simulink model "NewModuleTry_cs"  (Simulink 8.4)
settings: Solver=ode5  SolverMode=SingleTasking  StartTime=0.0  StopTime=inf  FixedStep=1/100  RelTol=1e-3
model workspace (MAT data in the model file):
  mbox_table : struct (value not decoded)
  model_closed = 0
  sim_status : num (value not decoded)
PreLoadFcn:
  | mbxruntime.callbacks.PreLoadFcn(bdroot);
PostLoadFcn:
  | mbxruntime.callbacks.PostLoadFcn(bdroot);
InitFcn:
  | mbxruntime.callbacks.InitFcn(bdroot);
StartFcn:
  | mbxruntime.callbacks.StartFcn(bdroot);
StopFcn:
  | mbxruntime.callbacks.StopFcn(bdroot);
undefined symbols (not defined in the file or in its folder): dfreq, gray, InitImageOutputDir, Rec, SDTV, strel
libraries: simulink x41, PreScanSimulinkLibrary x15, visiontextngfix x15, simulink_extras x12, visionconversions x3, PreScanUsefulBlocks x3, visionsinks x2, visionstatistics x1, visionmorphops x1, visionanalysis x1, simulink_need_slupdate x1
(part 1 of 7)
CloseFcn:
  | mbxruntime.callbacks.CloseFcn(bdroot);
settings Model: Creator=PRESCAN  LastModifiedBy=vj-admin
settings OptimizationCC: InitFltsAndDblsToZero=on
settings DebuggingCC: SaveWithParameterizedLinksMsg=none  SignalResolutionControl=TryResolveAllWithWarning  SolverPrmCheckMsg=none  MultiTaskDSMMsg=warning  MultiTaskCondExecSysMsg=none
settings ModelReferenceCC: UpdateModelReferenceTargets=IfOutOfDate
settings SFSimCC: SimParseCustomCode=off
settings SFSimCC: SimCustomHeaderCode=|
  | #include "prescan_collisiondetection_data.h"
  | #include "prescan.h"
  | #include "prescan_platform.h"
  | #include "prescan_v2x_data.h"
settings RTWCC: IncludeERTFirstTime=on
settings GRTTargetCC: TargetFcnLib=ansi_tfl_tmw.mat

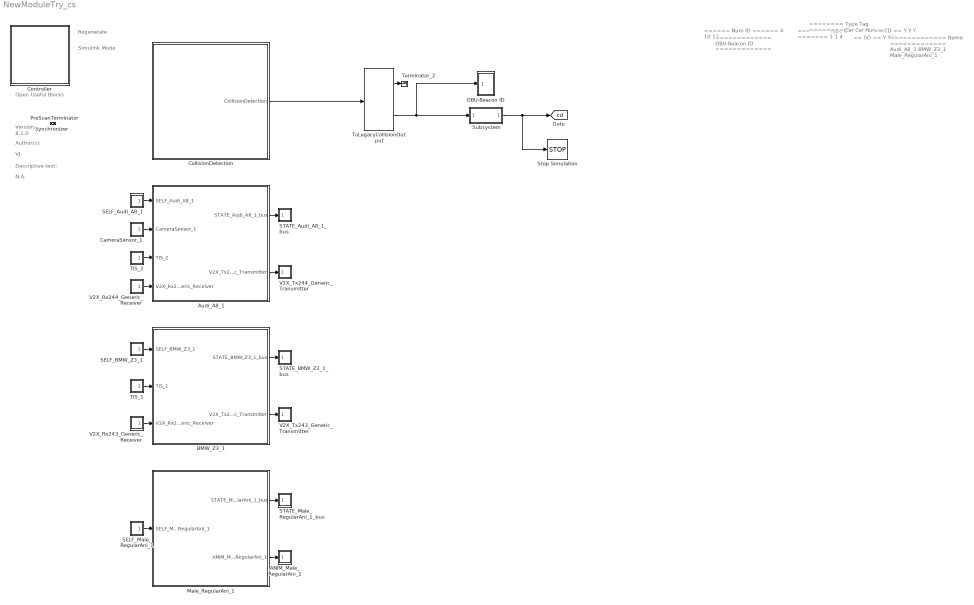
== system NewModuleTry_cs ==
  note: Regenerate
  note: Simulink Mode
  note: Open Useful Blocks
  note: 8.1.0
  note: Version:
  note: Author(s):
  note: VJ
  note: Descriptive text:
  note: N.A.
  note: ======
      | Num ID
      | ======
      | 4
      | 10
      | 11
  note: =============
      | OBU-Beacon ID
      | =============
  note: =======
      | Type ID
      | =======
      | 1
      | 1
      | 4
  note: ========
      | Type Tag
      | ========
      | Car
      | Car
      | Human
  note: ==
      | SD
      | ==
      | Y
      | Y
      | Y
  note: ==
      | CD
      | ==
      | Y
      | Y
      | Y
  note: =============
      | Name
      | =============
      | Audi_A8_1
      | BMW_Z3_1
      | Male_RegularAni_1
  ANIM_Male_RegularAni_1 : Subsystem  Tag=actuator/AnimationOutport  Priority=0  LoadFcn=load('PreScanAnimActuatorData.mat')  Variant=on  OverrideUsingVariant=on  mask(PreScan Sink Block: State Animation){}
      mask help: The Human Animation port allows the human to walk, run or bend
      settings: OpenFcn=open_system([gcb '/ENABLED/Actuator'],'mask')
      mask Help: eval('openHelp(239)')
      mask Display: image(imread('HumanAnimated.jpg'))
  Audi_A8_1 : Subsystem  Tag=WorldObjectSubSystem  InitFcn=UniqueId = '58';  Variant=on  OverrideUsingVariant=on
      mask init:
      | imagePath=which('Audi_A8.jpg');
      settings: OpenFcn=open_system([gcb '/ENABLED'])
      mask Display: image(imread(imagePath));color('white');text(0,0,' ID=4\n')
  BMW_Z3_1 : Subsystem  Tag=WorldObjectSubSystem  InitFcn=UniqueId = '59';  Variant=on  OverrideUsingVariant=on
      mask init:
      | imagePath=which('BMW_Z3.jpg');
      settings: OpenFcn=open_system([gcb '/ENABLED'])
      mask Display: image(imread(imagePath));color('white');text(0,0,' ID=10\n')
  CameraSensor_1 : Subsystem  Tag=sensor/Camera/CameraSensor  Priority=3  Variant=on  OverrideUsingVariant=on  mask(PreScan Source Block: Camera Sensor){}
      mask help: The Camera Sensor provides a color or monochrome image.
      settings: OpenFcn=open_system([gcb '/ENABLED/Sensor'],'mask')
      mask Help: eval('openHelp(457)')
      mask Display: image(imread('CameraSensor.png'))
  CollisionDetection : Subsystem  Tag=sensor/CollisionDetection  Priority=3  LoadFcn=load('PrescanCollisionDetectionData.mat');load('PrescanCollisionDetectionMessage.mat')  Variant=on  OverrideUsingVariant=on  mask(PreScan Source Block: CollisionDetection){}
      mask help: Collision Detection can be used to detect collisions between PreScan components. For Collision Detection the actual component shape is taken into account, so it is not a bounding box approach.
      settings: OpenFcn=open_system([gcb '/ENABLED/Sensor'],'mask')
      mask Help: eval('openHelp(811)')
      mask Display: image(imread('crash.jpg'))
  Controller : Subsystem  Description=A11229525821A304D5856380C190912EEAC74B144EF439124D49D263F028B97E  Priority=-1  LoadFcn=load PreScanControllerData  mask(PreScan Simulation Controller){prescanversion='8.1.0', ModelReferencing=off, TimeStep=1/100, ControlMode=0, PreScanExecutionMode=on, ControllerCount=0, ControllerIndex=0, ControllerOptions=''}
      mask prompts: prescanversion "PreScan Version"; ModelReferencing "Use Model Referencing"; TimeStep "Upload Period [s]"; ControlMode "Control Mode"; PreScanExecutionMode "Execution Mode"; ControllerCount "Controller Count"; ControllerIndex "Controller Index"; ControllerOptions "Controller Options"
      mask help:
      | Please do not remove this block from the compilation sheet,
      | as it connects the model to the PreScan environment.
      mask init:
      | model = bdroot(gcb);
      | ExperimentFile = mbxruntime.findExperimentFile(model);
      | 
      | [d1, d2, d3, prescandata] = prescan_Settings();
      | ModelDepo = fullfile(prescandata,'ModelDepo'); 
      | 
      | RTmode = 0;
      | actors = find_system(model,'SearchDepth', 1,'LookUnderMasks', 'all','Tag','WorldObjectSubSystem');
      | for ii=1:length(actors)
      |     actormode = get_param(actors{ii},'OverrideUsingVariant');
      |     if strcmpi(actormode,'off')
      |         RTmode = 1;
      |     end
      | end
      | 
      | SimulationMode = get_param(bdroot,'SimulationMode');
      | if strcmp(SimulationMode, 'rapid-accelerator')
      |     SimulationMode = 'external';
      | end
      | TargetName = get_param(bdroot,'SystemTargetFile');
      settings: ModelCloseFcn=assignin('base',['model_closed_' bdroot],true);
      mask Help: eval('openHelp(812)')
      mask Display: image(imread('prescanlogo.ico'))
  Male_RegularAni_1 : Subsystem  Tag=WorldObjectSubSystem  InitFcn=UniqueId = '60';  Variant=on  OverrideUsingVariant=on
      mask init:
      | imagePath=which('Male_RegularAni.jpg');
      settings: OpenFcn=open_system([gcb '/ENABLED'])
      mask Display: image(imread(imagePath));color('white');text(0,0,' ID=11\n')
  OBU-Beacon ID : Subsystem  Tag=Scope Collision Detections
      settings: DeleteFcn=PreScanBlockDeleteFcn;
      settings: OpenFcn=|
      | blockname=[get_param(gcb,'Parent'),'/',get_param(gcb,'Name')];
      | subblockname=[blockname,'/Collision Detections'];
      | open_system(subblockname);
      | close_system(blockname);
      mask Display:
      | plot([0.5 9.5 9.5 0.5 0.5],[5 5 9 9 5])
      | plot(0,0)
      | plot(10,10)
      | text(0,1,'P+')
  PreScanTerminator : Subsystem  Tag=PreScanTerminator  Priority=999  LoadFcn=load PrescanTerminatorData  mask(PreScan Simulation Terminator){TimeStep=1/100}
      mask prompts: TimeStep "Upload Period [s]"
      mask help:
      | Please do not remove this block from the compilation sheet as it
      | connects the model to the PreScan environment.
      mask Help: eval('openHelp(812)')
      mask Display: image(imread('prescanlogo.ico'))
  SELF_Audi_A8_1 : Subsystem  Tag=sensor/SelfPort  Priority=3  LoadFcn=load('PreScanSelfSensorData.mat')  Variant=on  OverrideUsingVariant=on  mask(PreScan Source Block: SELF){}
      mask help:
      | The SELF port shows (state) information of the actor itself. The outputs are position in the experiment's axis system and the GPS coordinates, and the object's absolute velocity and compass heading.
      |
      | For more information, please click Help.
      settings: OpenFcn=open_system([gcb '/ENABLED/Sensor'],'mask')
      mask Help: eval('openHelp(462)')
      mask Display: image(imread('GPS.png'))
  SELF_BMW_Z3_1 : Subsystem  Tag=sensor/SelfPort  Priority=3  LoadFcn=load('PreScanSelfSensorData.mat')  Variant=on  OverrideUsingVariant=on  mask(PreScan Source Block: SELF){}
      mask help:
      | The SELF port shows (state) information of the actor itself. The outputs are position in the experiment's axis system and the GPS coordinates, and the object's absolute velocity and compass heading.
      |
      | For more information, please click Help.
      settings: OpenFcn=open_system([gcb '/ENABLED/Sensor'],'mask')
      mask Help: eval('openHelp(462)')
      mask Display: image(imread('GPS.png'))
  SELF_Male_RegularAni_1 : Subsystem  Tag=sensor/SelfPort  Priority=3  LoadFcn=load('PreScanSelfSensorData.mat')  Variant=on  OverrideUsingVariant=on  mask(PreScan Source Block: SELF){}
      mask help:
      | The SELF port shows (state) information of the actor itself. The outputs are position in the experiment's axis system and the GPS coordinates, and the object's absolute velocity and compass heading.
      |
      | For more information, please click Help.
      settings: OpenFcn=open_system([gcb '/ENABLED/Sensor'],'mask')
      mask Help: eval('openHelp(462)')
      mask Display: image(imread('GPS.png'))
  STATE_Audi_A8_1_bus : Subsystem  Tag=actuator/StatePort  Priority=0  LoadFcn=load('PreScanStateActuatorData.mat')  Variant=on  OverrideUsingVariant=on  mask(PreScan Sink Block: State){}
      mask help:
      | The Actor State contains a vector signal of size (9x1), containing the following signals:
      |
      | -  Position    	(x,y,z)             	[m]
      | -  Velocity    	(vx,vy,vz)         	[m/s]
      | -  Angles       	(Roll, Pitch, Yaw)	[rad]
      |
      | The Actor state is defined in the global axis system.
      | The state is superponed on the Initial position defined in the GUI.
      |
      | For more information, please click Help.
      settings: OpenFcn=open_system([gcb '/ENABLED/Actuator'],'mask')
      mask Help: eval('openHelp(222)')
      mask Display: image(imread('State.png'))
  STATE_BMW_Z3_1_bus : Subsystem  Tag=actuator/StatePort  Priority=0  LoadFcn=load('PreScanStateActuatorData.mat')  Variant=on  OverrideUsingVariant=on  mask(PreScan Sink Block: State){}
      mask help:
      | The Actor State contains a vector signal of size (9x1), containing the following signals:
      |
      | -  Position    	(x,y,z)             	[m]
      | -  Velocity    	(vx,vy,vz)         	[m/s]
      | -  Angles       	(Roll, Pitch, Yaw)	[rad]
      |
      | The Actor state is defined in the global axis system.
      | The state is superponed on the Initial position defined in the GUI.
      |
      | For more information, please click Help.
      settings: OpenFcn=open_system([gcb '/ENABLED/Actuator'],'mask')
      mask Help: eval('openHelp(222)')
      mask Display: image(imread('State.png'))
  STATE_Male_RegularAni_1_bus : Subsystem  Tag=actuator/StatePort  Priority=0  LoadFcn=load('PreScanStateActuatorData.mat')  Variant=on  OverrideUsingVariant=on  mask(PreScan Sink Block: State){}
      mask help:
      | The Actor State contains a vector signal of size (9x1), containing the following signals:
      |
      | -  Position    	(x,y,z)             	[m]
      | -  Velocity    	(vx,vy,vz)         	[m/s]
      | -  Angles       	(Roll, Pitch, Yaw)	[rad]
      |
      | The Actor state is defined in the global axis system.
      | The state is superponed on the Initial position defined in the GUI.
      |
      | For more information, please click Help.
      settings: OpenFcn=open_system([gcb '/ENABLED/Actuator'],'mask')
      mask Help: eval('openHelp(222)')
      mask Display: image(imread('State.png'))
  Stop Simulation : Stop
  Subsystem : Subsystem
      mask Display: fprintf('CD');
  Synchronizer : Subsystem  Tag=PreScanSynchronizer  Priority=1  LoadFcn=load PrescanSynchronizeData  mask(PreScan Simulation Core Block){TimeStep=1/100}
      mask prompts: TimeStep "Timestep [s]"
      mask help:
      | Please do not remove this block from the PreScan compilation sheet,
      | as it contains essential configuration parameters for a PreScan simulation.
      settings: DeleteFcn=PreScanBlockDeleteFcn;
      mask Display: image(imread('prescanlogo.ico'))
  TIS_1 : Subsystem  Tag=sensor/TIS  Priority=3  LoadFcn=load('PrescanScannerSensorData.mat');load('PrescanScannerSensorMessage.mat')  Variant=on  OverrideUsingVariant=on  mask(PreScan Source Block: Technology Independent Sensor (TIS)){}
      mask help:
      | The Technology Independent Sensor (TIS) provides a sensor with all sensor-related influence factors (like noise, drift and accuracy) without being technology specific (like radar and lidar). The TIS detects the closest point on the geometry of an object.
      |
      | For more information, please click Help.
      settings: OpenFcn=open_system([gcb '/ENABLED/Sensor'],'mask')
      mask Help: eval('openHelp(449)')
      mask Display: image(imread('TIS.png'))
  TIS_2 : Subsystem  Tag=sensor/TIS  Priority=3  LoadFcn=load('PrescanScannerSensorData.mat');load('PrescanScannerSensorMessage.mat')  Variant=on  OverrideUsingVariant=on  mask(PreScan Source Block: Technology Independent Sensor (TIS)){}
      mask help:
      | The Technology Independent Sensor (TIS) provides a sensor with all sensor-related influence factors (like noise, drift and accuracy) without being technology specific (like radar and lidar). The TIS detects the closest point on the geometry of an object.
      |
      | For more information, please click Help.
      settings: OpenFcn=open_system([gcb '/ENABLED/Sensor'],'mask')
      mask Help: eval('openHelp(449)')
      mask Display: image(imread('TIS.png'))
  Terminator_2 : Terminator
  ToLegacyCollisionOutput : PreScanUsefulBlocks/ToLegacyCollisionOutput
  V2X_Rx243_Generic_Receiver : Subsystem  Tag=sensor/plugin/sfun_V2X_Generic_Receiver  Priority=3  Variant=on  OverrideUsingVariant=on  mask(V2X Generic Receiver Block){}
      mask help: V2X Block receiving a Generic message
      settings: OpenFcn=open_system([gcb '/ENABLED/Sensor'],'mask')
      mask Help: eval('openHelp()')
      mask Display: image(imread('V2XR_grayscale.png'))
  V2X_Rx244_Generic_Receiver : Subsystem  Tag=sensor/plugin/sfun_V2X_Generic_Receiver  Priority=3  Variant=on  OverrideUsingVariant=on  mask(V2X Generic Receiver Block){}
      mask help: V2X Block receiving a Generic message
      settings: OpenFcn=open_system([gcb '/ENABLED/Sensor'],'mask')
      mask Help: eval('openHelp()')
      mask Display: image(imread('V2XR_grayscale.png'))
  V2X_Tx243_Generic_Transmitter : Subsystem  Tag=actuator/plugin/sfun_V2X_Generic_Transmitter  Priority=0  Variant=on  OverrideUsingVariant=on  mask(V2X Generic Transmitter Block){}
      mask help: V2X Block transmitting a Generic message
      settings: OpenFcn=open_system([gcb '/ENABLED/Actuator'],'mask')
      mask Help: eval('openHelp()')
      mask Display: image(imread('V2XT_grayscale.png'))
  V2X_Tx244_Generic_Transmitter : Subsystem  Tag=actuator/plugin/sfun_V2X_Generic_Transmitter  Priority=0  Variant=on  OverrideUsingVariant=on  mask(V2X Generic Transmitter Block){}
      mask help: V2X Block transmitting a Generic message
      settings: OpenFcn=open_system([gcb '/ENABLED/Actuator'],'mask')
      mask Help: eval('openHelp()')
      mask Display: image(imread('V2XT_grayscale.png'))
  tag scope: cd=global
  wires:
  CollisionDetection/1(CollisionDetection) -> ToLegacyCollisionOutput/1
  Subsystem/1(cd_out) -> Stop Simulation/1, [cd]
  ToLegacyCollisionOutput/2 -> Subsystem/1(cd_in), OBU-Beacon ID/1(In1)
  ToLegacyCollisionOutput/1 -> Terminator_2/1
  Audi_A8_1/1(STATE_Audi_A8_1_bus) -> STATE_Audi_A8_1_bus/1(STATE_Audi_A8_1_bus)
  SELF_Audi_A8_1/1(SELF_Audi_A8_1) -> Audi_A8_1/1(SELF_Audi_A8_1)
  CameraSensor_1/1(CameraSensor_1) -> Audi_A8_1/2(CameraSensor_1)
  TIS_2/1(TIS_2) -> Audi_A8_1/3(TIS_2)
  Audi_A8_1/2(V2X_Tx244_Generic_Transmitter) -> V2X_Tx244_Generic_Transmitter/1(V2X_Tx244_Generic_Transmitter)
  V2X_Rx244_Generic_Receiver/1(V2X_Rx244_Generic_Receiver) -> Audi_A8_1/4(V2X_Rx244_Generic_Receiver)
  BMW_Z3_1/1(STATE_BMW_Z3_1_bus) -> STATE_BMW_Z3_1_bus/1(STATE_BMW_Z3_1_bus)
  SELF_BMW_Z3_1/1(SELF_BMW_Z3_1) -> BMW_Z3_1/1(SELF_BMW_Z3_1)
  TIS_1/1(TIS_1) -> BMW_Z3_1/2(TIS_1)
  BMW_Z3_1/2(V2X_Tx243_Generic_Transmitter) -> V2X_Tx243_Generic_Transmitter/1(V2X_Tx243_Generic_Transmitter)
  V2X_Rx243_Generic_Receiver/1(V2X_Rx243_Generic_Receiver) -> BMW_Z3_1/3(V2X_Rx243_Generic_Receiver)
  Male_RegularAni_1/1(STATE_Male_RegularAni_1_bus) -> STATE_Male_RegularAni_1_bus/1(STATE_Male_RegularAni_1_bus)
  Male_RegularAni_1/2(ANIM_Male_RegularAni_1) -> ANIM_Male_RegularAni_1/1(ANIM_Male_RegularAni_1)
  SELF_Male_RegularAni_1/1(SELF_Male_RegularAni_1) -> Male_RegularAni_1/1(SELF_Male_RegularAni_1)

== system NewModuleTry_cs/ANIM_Male_RegularAni_1 ==
  ANIM_Male_RegularAni_1 : Inport  Tag=inport/AnimationOutport  OutDataTypeStr=Bus: PRESCAN_ANIMACTUATORDATA  PortDimensions=1  SampleTime=1/100  BusOutputAsStruct=on
  DISABLED : Subsystem  VariantControl=off
  ENABLED : Subsystem  VariantControl=on

== system NewModuleTry_cs/Audi_A8_1 ==
  SELF_Audi_A8_1 : Inport  Tag=inport/SelfPort  OutDataTypeStr=Bus: PRESCAN_SELFSENSORDATA  PortDimensions=1  SampleTime=1/100  BusOutputAsStruct=on
  CameraSensor_1 : Inport  Tag=inport/Camera/CameraSensor  Port=2  OutDataTypeStr=uint8  SampleTime=1/50  BusOutputAsStruct=on
  TIS_2 : Inport  Tag=inport/TIS  Port=3  OutDataTypeStr=Bus: PRESCAN_SCANNERSENSOR_MESSAGE  PortDimensions=1  SampleTime=1/25  BusOutputAsStruct=on
  V2X_Rx244_Generic_Receiver : Inport  Tag=inport/plugin/sfun_V2X_Generic_Receiver  Port=4  BusOutputAsStruct=on
  DISABLED : Subsystem  VariantControl=off
  ENABLED : Subsystem  VariantControl=on
  STATE_Audi_A8_1_bus : Outport  Tag=outport/StatePort  OutDataTypeStr=Bus: PRESCAN_STATEACTUATORDATA  PortDimensions=1  SampleTime=1/100
  V2X_Tx244_Generic_Transmitter : Outport  Tag=outport/plugin/sfun_V2X_Generic_Transmitter  Port=2

== system NewModuleTry_cs/BMW_Z3_1 ==
  SELF_BMW_Z3_1 : Inport  Tag=inport/SelfPort  OutDataTypeStr=Bus: PRESCAN_SELFSENSORDATA  PortDimensions=1  SampleTime=1/100  BusOutputAsStruct=on
  TIS_1 : Inport  Tag=inport/TIS  Port=2  OutDataTypeStr=Bus: PRESCAN_SCANNERSENSOR_MESSAGE  PortDimensions=1  SampleTime=1/25  BusOutputAsStruct=on
  V2X_Rx243_Generic_Receiver : Inport  Tag=inport/plugin/sfun_V2X_Generic_Receiver  Port=3  BusOutputAsStruct=on
  DISABLED : Subsystem  VariantControl=off
  ENABLED : Subsystem  VariantControl=on
  STATE_BMW_Z3_1_bus : Outport  Tag=outport/StatePort  OutDataTypeStr=Bus: PRESCAN_STATEACTUATORDATA  PortDimensions=1  SampleTime=1/100
  V2X_Tx243_Generic_Transmitter : Outport  Tag=outport/plugin/sfun_V2X_Generic_Transmitter  Port=2

== system NewModuleTry_cs/CameraSensor_1 ==
  DISABLED : Subsystem  VariantControl=off
  ENABLED : Subsystem  VariantControl=on
  CameraSensor_1 : Outport  Tag=outport/Camera/CameraSensor  OutDataTypeStr=uint8  SampleTime=1/50

== system NewModuleTry_cs/CollisionDetection ==
  DISABLED : Subsystem  VariantControl=off
  ENABLED : Subsystem  VariantControl=on
  CollisionDetection : Outport  Tag=outport/CollisionDetection  OutDataTypeStr=Bus: PRESCAN_COLLISIONDETECTION_MESSAGE  PortDimensions=1  SampleTime=1/100

== system NewModuleTry_cs/Controller ==
  Terminator : Terminator
  sfun_Controller : S-Function  FunctionName=sfun_Controller  Parameters=SParameter1, SParameter2, SParameter3, SParameter4, SParameter5, SParameter6, SParameter7, SParameter8, SParameter9, SParameter10, SampleTime  EnableBusSupport=off  mask(Legacy Function){SFunctionSpec=void prescan_outputFcn(void** work1, PRESCAN_CONTROLLERDATA y1[1]), SParameter1=uint8([ExperimentFile 0]), SParameter2=uint8([ModelDepo 0]), SParameter3=uint8([ControllerOptions 0]), SParameter4=RTmode, SParameter5=PreScanExecutionMode, SParameter6=ControlMode, SParameter7=ControllerCount, SParameter8=ControllerIndex, SParameter9=uint8([SimulationMode 0]), SParameter10=uint8([TargetName 0]), SampleTime=TimeStep, ShowSpec=on}
      mask prompts: SParameter1 "P1:"; SParameter2 "P2:"; SParameter3 "P3:"; SParameter4 "P4:"; SParameter5 "P5:"; SParameter6 "P6:"; SParameter7 "P7:"; SParameter8 "P8:"; SParameter9 "P9:"; SParameter10 "P10:"; SampleTime "Sample time (-1 for inherited):"; ShowSpec "Display function specification"
      mask help:
      | This block allows you to call the legacy functions specified by the following Legacy Code Tool definition:
      | def.SFunctionName = 'sfun_Controller';
      | def.OutputFcnSpec = 'void prescan_outputFcn(void** work1, PRESCAN_CONTROLLERDATA y1[1])';
      | def.StartFcnSpec = 'void prescan_startFcn(void ** work1, uint8 p1[], uint8 p2[], uint8 p3[], double p4, double p5, double p6, double p7, double p8, uint8 p9[], uint8 p10[])';
      | def.TerminateFcnSpec = 'void prescan_terminateFcn(void** work1)';
      | def.HeaderFiles = {'prescan_controller_data.h', 'prescan_SFunLibrary.h', 'prescan_LogHandler.h', 'prescan_CreateLogHandler.h', 'prescan_ErrorHandler.h', 'prescan_CreateErrorHandler.h', 'prescan_modify.h', 'ModuleDLL.h'};
      | def.SourceFiles = {'prescan_MexLogHandler.cpp', 'prescan_SimStructErrorHandler.cpp', 'prescan_LogHandler.cpp', 'prescan_ErrorHandler.cpp', 'prescan_Modify.cpp'};
      | def.HostLibFiles = {'sensorinterfaced.lib'};
      | def.TargetLibFiles = {'sensorinterfaced.so'};
      | def.IncPaths = {'.', 'C:\projects\prescan\rt_vislibrary\vis\..\pimp\include\sensors\InterfaceRTW'};
      | def.SrcPaths = {'C:\projects\prescan\rt_vislibrary\vis\..\pimp\include\sensors\InterfaceRTW', 'C:\projects\prescan\rt_vislibrary\vis\..\pimp\include\sensors\InterfaceRTW\ccurrt'};
      | def.LibPaths = {'C:\\projects\\prescan\\vislibrary_build\lib'};
      | def.SampleTime = 'parameterized';
      mask Help: <p>This block was generated automatically by the Legacy Code Tool. For detailed help on this tool, call<a href="matlab:legacy_code('help')"> legacy_code('help')</a>.</p>
      mask Callback ShowSpec:
      | if strcmp(get_param(gcbh, 'ShowSpec'), 'on')
      |   set_param(gcbh, 'MaskDisplay', sprintf('fprintf(''%s'');', get_param(gcbh, 'SFunctionSpec')));
      | else
      |   set_param(gcbh, 'MaskDisplay', sprintf('fprintf(''%s'');', get_param(gcbh, 'FunctionName')));
      | end
      mask Display: fprintf('void prescan_outputFcn(void** work1, PRESCAN_CONTROLLERDATA y1[1])');
  wires:
  sfun_Controller/1 -> Terminator/1

== system NewModuleTry_cs/Male_RegularAni_1 ==
  SELF_Male_RegularAni_1 : Inport  Tag=inport/SelfPort  OutDataTypeStr=Bus: PRESCAN_SELFSENSORDATA  PortDimensions=1  SampleTime=1/100  BusOutputAsStruct=on
  DISABLED : Subsystem  VariantControl=off
  ENABLED : Subsystem  VariantControl=on
  STATE_Male_RegularAni_1_bus : Outport  Tag=outport/StatePort  OutDataTypeStr=Bus: PRESCAN_STATEACTUATORDATA  PortDimensions=1  SampleTime=1/100
  ANIM_Male_RegularAni_1 : Outport  Tag=outport/AnimationOutport  Port=2  OutDataTypeStr=Bus: PRESCAN_ANIMACTUATORDATA  PortDimensions=1  SampleTime=1/100

== system NewModuleTry_cs/OBU-Beacon ID ==
  In1 : Inport
  Collision Detections : Scope  NumInputPorts=5
      settings: YMin=0~0~0~0~0  YMax=10~10~10~10~10  SaveName=ScopeData2
  Demux2 : Demux  Outputs=5
  wires:
  In1/1 -> Demux2/1
  Demux2/5 -> Collision Detections/5
  Demux2/4 -> Collision Detections/4
  Demux2/3 -> Collision Detections/3
  Demux2/2 -> Collision Detections/2
  Demux2/1 -> Collision Detections/1

== system NewModuleTry_cs/PreScanTerminator ==
  Terminator : Terminator
  sfun_Terminator : S-Function  FunctionName=sfun_Terminator  Parameters=SampleTime  EnableBusSupport=off  mask(Legacy Function){SFunctionSpec=void prescan_terminator_outputFcn(void ** work1, PRESCAN_TERMINATORDATA y1[1]), SampleTime=TimeStep, ShowSpec=on}
      mask prompts: SampleTime "Sample time (-1 for inherited):"; ShowSpec "Display function specification"
      mask help:
      | This block allows you to call the legacy functions specified by the following Legacy Code Tool definition:
      | def.SFunctionName = 'sfun_Terminator';
      | def.OutputFcnSpec = 'void prescan_terminator_outputFcn(void ** work1, PRESCAN_TERMINATORDATA y1[1])';
      | def.StartFcnSpec = 'void prescan_terminator_startFcn(void ** work1)';
      | def.TerminateFcnSpec = 'void prescan_terminator_terminateFcn(void ** work1)';
      | def.HeaderFiles = {'prescan_terminator_data.h'};
      | def.HostLibFiles = {'sensorinterfaced.lib'};
      | def.IncPaths = {'src', 'C:\prescandev\vislibrary\vis\..\pimp\include\sensors\InterfaceRTW'};
      | def.SrcPaths = {'src'};
      | def.LibPaths = {'C:\\prescandev\\vislibrary_build\lib'};
      | def.SampleTime = 'parameterized';
      | def.Options.language = 'C++';
      mask Help: <p>This block was generated automatically by the Legacy Code Tool. For detailed help on this tool, call<a href="matlab:legacy_code('help')"> legacy_code('help')</a>.</p>
      mask Callback ShowSpec:
      | if strcmp(get_param(gcbh, 'ShowSpec'), 'on')
      |   set_param(gcbh, 'MaskDisplay', sprintf('fprintf(''%s'');', get_param(gcbh, 'SFunctionSpec')));
      | else
      |   set_param(gcbh, 'MaskDisplay', sprintf('fprintf(''%s'');', get_param(gcbh, 'FunctionName')));
      | end
      mask Display: fprintf('void prescan_terminator_outputFcn(void ** work1, PRESCAN_TERMINATORDATA y1[1])');
  wires:
  sfun_Terminator/1 -> Terminator/1

== system NewModuleTry_cs/SELF_Audi_A8_1 ==
  DISABLED : Subsystem  VariantControl=off
  ENABLED : Subsystem  VariantControl=on
  SELF_Audi_A8_1 : Outport  Tag=outport/SelfPort  OutDataTypeStr=Bus: PRESCAN_SELFSENSORDATA  PortDimensions=1  SampleTime=1/100

== system NewModuleTry_cs/SELF_BMW_Z3_1 ==
  DISABLED : Subsystem  VariantControl=off
  ENABLED : Subsystem  VariantControl=on
  SELF_BMW_Z3_1 : Outport  Tag=outport/SelfPort  OutDataTypeStr=Bus: PRESCAN_SELFSENSORDATA  PortDimensions=1  SampleTime=1/100

== system NewModuleTry_cs/SELF_Male_RegularAni_1 ==
  DISABLED : Subsystem  VariantControl=off
  ENABLED : Subsystem  VariantControl=on
  SELF_Male_RegularAni_1 : Outport  Tag=outport/SelfPort  OutDataTypeStr=Bus: PRESCAN_SELFSENSORDATA  PortDimensions=1  SampleTime=1/100

== system NewModuleTry_cs/STATE_Audi_A8_1_bus ==
  STATE_Audi_A8_1_bus : Inport  Tag=inport/StatePort  OutDataTypeStr=Bus: PRESCAN_STATEACTUATORDATA  PortDimensions=1  SampleTime=1/100  BusOutputAsStruct=on
  DISABLED : Subsystem  VariantControl=off
  ENABLED : Subsystem  VariantControl=on

== system NewModuleTry_cs/STATE_BMW_Z3_1_bus ==
  STATE_BMW_Z3_1_bus : Inport  Tag=inport/StatePort  OutDataTypeStr=Bus: PRESCAN_STATEACTUATORDATA  PortDimensions=1  SampleTime=1/100  BusOutputAsStruct=on
  DISABLED : Subsystem  VariantControl=off
  ENABLED : Subsystem  VariantControl=on

== system NewModuleTry_cs/STATE_Male_RegularAni_1_bus ==
  STATE_Male_RegularAni_1_bus : Inport  Tag=inport/StatePort  OutDataTypeStr=Bus: PRESCAN_STATEACTUATORDATA  PortDimensions=1  SampleTime=1/100  BusOutputAsStruct=on
  DISABLED : Subsystem  VariantControl=off
  ENABLED : Subsystem  VariantControl=on

== system NewModuleTry_cs/Subsystem ==
  cd_in : Inport
  Integer Delay : Delay  DelayLength=1  InputProcessing=Inherited
  Logical Operator : Logic  AllPortsSameDT=off  OutDataTypeStr=boolean
  cd_out : Outport
  wires:
  cd_in/1 -> Integer Delay/1, Logical Operator/1
  Logical Operator/1 -> cd_out/1
  Integer Delay/1 -> Logical Operator/2

== system NewModuleTry_cs/Synchronizer ==
  Bus Selector1 : BusSelector  OutputSignals=FederateStopped
  Stop Simulation : Stop
  sfun_Synchronizer : S-Function  FunctionName=sfun_Synchronizer  Parameters=SampleTime  EnableBusSupport=off  mask(Legacy Function){SFunctionSpec=void prescan_synchronizer_outputFcn(void ** work1, PRESCAN_SYNCHRONIZEDATA y1[1]), SampleTime=TimeStep, ShowSpec=on}
      mask prompts: SampleTime "Sample time (-1 for inherited):"; ShowSpec "Display function specification"
      mask help:
      | This block allows you to call the legacy functions specified by the following Legacy Code Tool definition:
      | def.SFunctionName = 'sfun_Synchronizer';
      | def.OutputFcnSpec = 'void prescan_synchronizer_outputFcn(void ** work1, PRESCAN_SYNCHRONIZEDATA y1[1])';
      | def.StartFcnSpec = 'void prescan_synchronizer_startFcn(void ** work1)';
      | def.TerminateFcnSpec = 'void prescan_synchronizer_terminateFcn(void ** work1)';
      | def.HeaderFiles = {'prescan_synchronizer_data.h'};
      | def.HostLibFiles = {'sensorinterfaced.lib'};
      | def.IncPaths = {'src', 'C:\prescandev\vislibrary\vis\..\pimp\include\sensors\InterfaceRTW'};
      | def.SrcPaths = {'src'};
      | def.LibPaths = {'C:\\prescandev\\vislibrary_build\lib'};
      | def.SampleTime = 'parameterized';
      | def.Options.language = 'C++';
      mask Help: <p>This block was generated automatically by the Legacy Code Tool. For detailed help on this tool, call<a href="matlab:legacy_code('help')"> legacy_code('help')</a>.</p>
      mask Callback ShowSpec:
      | if strcmp(get_param(gcbh, 'ShowSpec'), 'on')
      |   set_param(gcbh, 'MaskDisplay', sprintf('fprintf(''%s'');', get_param(gcbh, 'SFunctionSpec')));
      | else
      |   set_param(gcbh, 'MaskDisplay', sprintf('fprintf(''%s'');', get_param(gcbh, 'FunctionName')));
      | end
      mask Display: fprintf('void prescan_synchronizer_outputFcn(void ** work1, PRESCAN_SYNCHRONIZEDATA y1[1])');
  wires:
  Bus Selector1/1 -> Stop Simulation/1  "<FederateStopped>"
  sfun_Synchronizer/1 -> Bus Selector1/1

== system NewModuleTry_cs/TIS_1 ==
  DISABLED : Subsystem  VariantControl=off
  ENABLED : Subsystem  VariantControl=on
  TIS_1 : Outport  Tag=outport/TIS  OutDataTypeStr=Bus: PRESCAN_SCANNERSENSOR_MESSAGE  PortDimensions=1  SampleTime=1/25

== system NewModuleTry_cs/TIS_2 ==
  DISABLED : Subsystem  VariantControl=off
  ENABLED : Subsystem  VariantControl=on
  TIS_2 : Outport  Tag=outport/TIS  OutDataTypeStr=Bus: PRESCAN_SCANNERSENSOR_MESSAGE  PortDimensions=1  SampleTime=1/25

== system NewModuleTry_cs/V2X_Rx243_Generic_Receiver ==
  DISABLED : Subsystem  VariantControl=off
  ENABLED : Subsystem  VariantControl=on
  V2X_Rx243_Generic_Receiver : Outport  Tag=outport/plugin/sfun_V2X_Generic_Receiver

== system NewModuleTry_cs/V2X_Rx244_Generic_Receiver ==
  DISABLED : Subsystem  VariantControl=off
  ENABLED : Subsystem  VariantControl=on
  V2X_Rx244_Generic_Receiver : Outport  Tag=outport/plugin/sfun_V2X_Generic_Receiver

== system NewModuleTry_cs/V2X_Tx243_Generic_Transmitter ==
  V2X_Tx243_Generic_Transmitter : Inport  Tag=inport/plugin/sfun_V2X_Generic_Transmitter  BusOutputAsStruct=on
  DISABLED : Subsystem  VariantControl=off
  ENABLED : Subsystem  VariantControl=on

== system NewModuleTry_cs/V2X_Tx244_Generic_Transmitter ==
  V2X_Tx244_Generic_Transmitter : Inport  Tag=inport/plugin/sfun_V2X_Generic_Transmitter  BusOutputAsStruct=on
  DISABLED : Subsystem  VariantControl=off
  ENABLED : Subsystem  VariantControl=on

== system NewModuleTry_cs/ANIM_Male_RegularAni_1/DISABLED ==
  ANIM_Male_RegularAni_1 : Inport  Tag=inport/AnimationOutport  OutDataTypeStr=Bus: PRESCAN_ANIMACTUATORDATA  PortDimensions=1  SampleTime=1/100  BusOutputAsStruct=on
  TRM1 : Terminator
  wires:
  ANIM_Male_RegularAni_1/1 -> TRM1/1

== system NewModuleTry_cs/ANIM_Male_RegularAni_1/ENABLED ==
  ANIM_Male_RegularAni_1 : Inport  Tag=inport/AnimationOutport  OutDataTypeStr=Bus: PRESCAN_ANIMACTUATORDATA  PortDimensions=1  SampleTime=1/100  BusOutputAsStruct=on
  Actuator : S-Function  FunctionName=sfun_AnimActuator  Parameters=UniqueID, TimeStep  EnableBusSupport=off  mask(PreScan Sink Block: State Animation){UniqueID=60, TimeStep=1/100}
      mask prompts: UniqueID "Auto-Assigned: Unique ID"; TimeStep "Auto-Assigned: Upload Period [s]"
      mask help: The Human Animation port allows the human to walk, run or bend
      mask Help: eval('openHelp(239)')
      mask Display: image(imread('HumanAnimated.jpg'))
  wires:
  ANIM_Male_RegularAni_1/1 -> Actuator/1

== system NewModuleTry_cs/Audi_A8_1/DISABLED ==
  SELF_Audi_A8_1 : Inport  Tag=inport/SelfPort  OutDataTypeStr=Bus: PRESCAN_SELFSENSORDATA  PortDimensions=1  SampleTime=1/100  BusOutputAsStruct=on
  CameraSensor_1 : Inport  Tag=inport/Camera/CameraSensor  Port=2  OutDataTypeStr=uint8  SampleTime=1/50  BusOutputAsStruct=on
  TIS_2 : Inport  Tag=inport/TIS  Port=3  OutDataTypeStr=Bus: PRESCAN_SCANNERSENSOR_MESSAGE  PortDimensions=1  SampleTime=1/25  BusOutputAsStruct=on
  V2X_Rx244_Generic_Receiver : Inport  Tag=inport/plugin/sfun_V2X_Generic_Receiver  Port=4  BusOutputAsStruct=on
  GND1 : Subsystem
  GND2 : Ground
  TRM{1..4} (4 alike) : Terminator
  STATE_Audi_A8_1_bus : Outport  Tag=outport/StatePort  OutDataTypeStr=Bus: PRESCAN_STATEACTUATORDATA  PortDimensions=1  SampleTime=1/100
  V2X_Tx244_Generic_Transmitter : Outport  Tag=outport/plugin/sfun_V2X_Generic_Transmitter  Port=2
  wires:
  SELF_Audi_A8_1/1 -> TRM1/1
  CameraSensor_1/1 -> TRM2/1
  TIS_2/1 -> TRM3/1
  V2X_Rx244_Generic_Receiver/1 -> TRM4/1
  GND1/1(bus) -> STATE_Audi_A8_1_bus/1
  GND2/1 -> V2X_Tx244_Generic_Transmitter/1

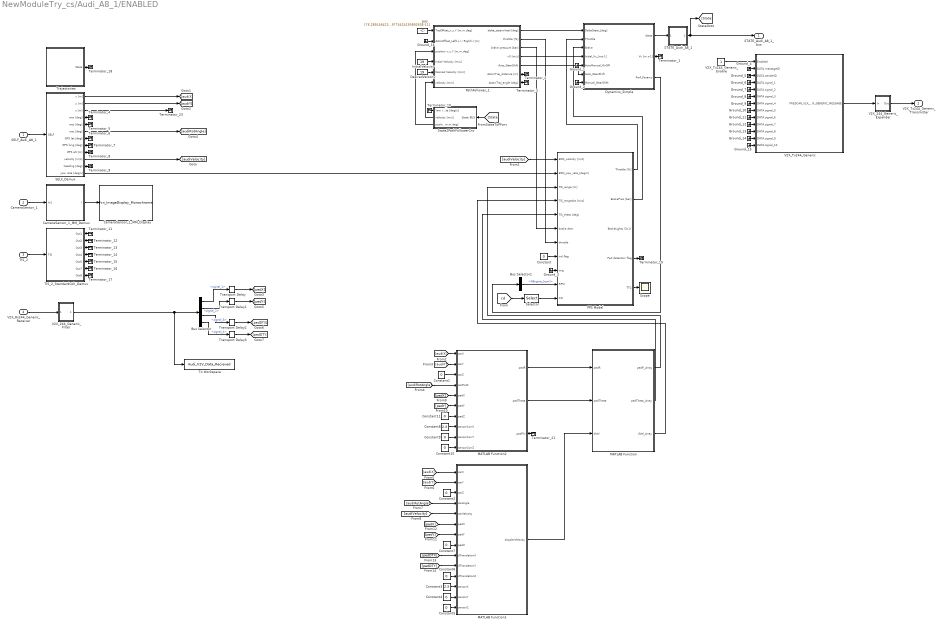
== system NewModuleTry_cs/Audi_A8_1/ENABLED ==
  SELF_Audi_A8_1 : Inport  Tag=inport/SelfPort  OutDataTypeStr=Bus: PRESCAN_SELFSENSORDATA  PortDimensions=1  SampleTime=1/100  BusOutputAsStruct=on
  CameraSensor_1 : Inport  Tag=inport/Camera/CameraSensor  Port=2  OutDataTypeStr=uint8  SampleTime=1/50  BusOutputAsStruct=on
  TIS_2 : Inport  Tag=inport/TIS  Port=3  OutDataTypeStr=Bus: PRESCAN_SCANNERSENSOR_MESSAGE  PortDimensions=1  SampleTime=1/25  BusOutputAsStruct=on
  V2X_Rx244_Generic_Receiver : Inport  Tag=inport/plugin/sfun_V2X_Generic_Receiver  Port=4  BusOutputAsStruct=on
  Bus Selector : BusSelector  OutputSignals=DATA.signal_1,DATA.signal_2,DATA.signal_3,DATA.signal_4
  Bus Selector1 : BusSelector  OutputSignals=NEngine_[rpm]
  CameraSensor_1_MM_Demux : Subsystem  Tag=demux/Camera/Monochrome  mask{SensorName=CameraSensor_1, hres=500, vres=375}
      mask prompts: SensorName "Sensor Name"; hres "Horizontal Resolution"; vres "Vertical Resolution"
      mask Help: eval('openHelp(457)')
      mask Display:
      | fprintf('MONO CAMERA:\n Monochrome\n %s \n %d x %d px',SensorName,hres,vres)
      | port_label('output',1,'I')
  CameraSensor_1_MM_Display : M-S-Function  Tag=CameraSensor_Monochrome_Display  InitFcn=InitImageOutputDir(gcb);  FunctionName=fcn_ImageDisplay_Monochrome  Parameters=SensorName EnableDisplay EnablePosition DisplayPosition FigureHandle SaveResults BitmapFormat TempOutputDir CameraType DataType  mask(PreScan Monochrome Display Block){SensorName=CameraSensor_1, EnableDisplay=on, EnablePosition=off, DisplayPosition=[10 10 500 375], FigureHandle=5801, SaveResults=off, Format=PNG, TempOutputDir=0, CameraType=Mono, DataType=uint8}
      mask prompts: SensorName "User Specified: Title of Display"; EnableDisplay "Active"; EnablePosition "Set Display window position"; DisplayPosition "Display window position [xpos ypos width height]"; FigureHandle "Unique handle"; SaveResults "Save results"; TempOutputDir "OutputDir"; CameraType "Camera Type"; DataType "Image Data Type"
      mask help: This block displays the Monochrome output of a PreScan camera sensor.
      mask init:
      | if EnableDisplay
      |     EnableString='';
      |     EnableColor='gray';
      | else
      |     EnableString='INACTIVE';
      |     EnableColor='red';
      | end
      | switch Format
      |     case 1
      |         BitmapFormat = 'png';
      |     case 2
      |         BitmapFormat = 'bmp';
      |     case 3
      |         BitmapFormat = 'jpg';
      | end
      | if CameraType==1
      |     CameraTypeName='MONO';
      |     PortNumber=0;
      | else
      |     CameraTypeName='STEREO';
      |     PortNumber=1;
      | end
      settings: CopyFcn=CopyFcnDisplay  DeleteFcn=PreScanBlockDeleteFcn;  ModelCloseFcn=fcn_ImageDisplay_ModelCloseFcn
      mask Help: eval('openHelp(457)')
      mask Callback EnablePosition:
      | MV=get_param(gcb,'MaskVisibilities');
      | if strcmp(get_param(gcb,'EnablePosition'),'on')
      |     MV{4}='on';
      | else
      |     MV{4}='off';
      | end
      | set_param(gcb,'MaskVisibilities',MV);
      | clear MV;
      mask TypeOptions Format: PNG | BMP | JPG
      mask TypeOptions CameraType: Mono | Stereo
      mask TypeOptions DataType: uint8 | single
      mask Display:
      | color(EnableColor);
      | fprintf('%s\n DISPLAY:\n Monochrome\n %s',EnableString,SensorName)
      | port_label('input',1,'I')
      | port_label('input',PortNumber+1,'I')
  Constant{,1..2,4..7,9..11} (10 alike) : Constant  Value=0
  Constant3 : Constant  Value=2.3
  Constant8 : Constant  Value=2.3
  DesiredVelocity : Constant  Tag=DesiredVelocity  Value=19
  Dynamics_Simple : Subsystem  Tag=Simple_Vehicle_Dynamics  mask(PreScan Block: Simple Dynamics){Migrate=on, TimeStep=1/100, ComputationMode=Continuous_Time}
      mask prompts: Migrate "Migrate. During migration this block will be replaced by a newer one."; TimeStep "Auto assigned: Time Step [s]"; ComputationMode "Computation mode:"
      mask help:
      | The Simple Dynamics Model is selected in the GUI to simulate vehicle dynamics behavior.
      |
      | The Simple Dynamics Model is completely open to the user. The parameters of this model can be set in the Simple Dynamics dialog in the GUI.
      |
      | For more information, please click Help.
      mask init:
      | p = SimpleDyn_pars;
      settings: DeleteFcn=PreScanBlockDeleteFcn;
      mask Help: eval('openHelp(220)')
      mask Display:
      | image(imread('SimpleDyn.png'))
      | port_label('input', 1, '{\delta}_S_t_ _e_e_r [deg]','texmode','on')
      | port_label('input', 2, 'Throttle [%]')
      | port_label('input', 3, 'Brake Pres [bar]')
      | port_label('input', 4, 'V_0 [ms-1]','texmode','on')
      | port_label('input', 5, 'Auto=[0]/Manual=[1]')
      | port_label('input', 6, 'Auto_GearShift')
      | port_label('input', 7, 'Manual_GearShift')
      | port_label('output', 1, 'State')
      | port_label('output', 2, 'Vx [ms-1]')
      | port_label('output', 3, 'Perf Params')
  Ground_{1..16} (16 alike) : Ground
  InitialVelocity : Constant  Tag=InitialVelocity  Value=19
  MATLAB Function : MATLAB Function  TreatAsAtomicUnit=on
  MATLAB Function1 : MATLAB Function  TreatAsAtomicUnit=on
  MATLAB Function2 : MATLAB Function  TreatAsAtomicUnit=on
  PPS Model : Subsystem  mask(PPS Model){MaxSpeed=70, MaxBrakePressure=150, BrakeDelay=100, LaneWidth=3.5, TISMaxRange=40, TISMaxTheta=60, TISfreq=25, TISdet=32, Camfreq=50, Mainfreq=100, DisplaySwitch=on, DisplayFreq=25, RadarSwitch=on, RadarFreq=25}
      mask prompts: MaxSpeed "Vehicle cut-off speed [km/h]"; MaxBrakePressure "Maximum value of braking pressure available [bar]"; BrakeDelay "Braking system delay [ms]"; LaneWidth "Lane width [m]"; TISMaxRange "TIS maximum range [m]"; TISMaxTheta "TIS maximum theta [deg]"; TISfreq "TIS frequency [Hz]"; TISdet "Max. number of Radar detected objects [-]"; Camfreq "Camera frequency [Hz]"; Mainfreq "Compilation sheet frequency [Hz]"; DisplaySwitch "Show EGO parameters visualization"; DisplayFreq "EGO parameters visualization frequency [Hz]"; RadarSwitch "Show radar visualization"; RadarFreq "Radar frequency [Hz]"
      mask help: PreScan Experiment and Pedestrian Protection System parameters
      mask Help: eval('openHelp(8130)')
      mask Callback DisplaySwitch:
      | en = get_param(gcb,'MaskEnables');
      | switch get_param(gcb, 'DisplaySwitch')
      |     case 'off'
      |         en{12} = 'off';
      |     case 'on'
      |         en{12} = 'on';
      | end
      | set_param(gcb,'MaskEnables',en);
      mask Callback RadarSwitch:
      | en = get_param(gcb,'MaskEnables');
      | switch get_param(gcb, 'RadarSwitch')
      |     case 'off'
      |         en{14} = 'off';
      |     case 'on'
      |         en{14} = 'on';
      | end
      | set_param(gcb,'MaskEnables',en);
  PathFollower_1 : Subsystem  Tag=pathFollower  mask(PreScan Block: Path Follower){Migrate=on, FileName='Trajectory_1.mat', TunableSteeringGain=1, XShifting_wrt_COG=0}
      mask prompts: Migrate "Migrate. During migration this block will be replaced by a newer one."; FileName "Trajectory Name"; TunableSteeringGain "TunableSteeringGain [-]"; XShifting_wrt_COG "XShifting_wrt_COG [m]"
      mask help:
      | The Path Follower Model is selected in the GUI to simulate driver behavior.
      |
      | For more information, please click Help.
      mask init:
      | load(['trajectories/',eval(FileName)])
      | traject=trajectory';
      | 
      | Traj_x=traject(:,2);
      | Traj_y=traject(:,3);
      | Traj_z=traject(:,4);
      | Traj_vx=traject(:,8);
      | Traj_vy=traject(:,9);
      | Traj_vz=traject(:,10);
      mask Help: eval('openHelp(232)')
  SELF_Demux : Subsystem  Tag=demux/SelfPort  mask(PreScan Demux Block:){}
      mask help:
      | The SELF port shows (state) information of the actor itself. The outputs are position in the experiment's axis system and the GPS coordinates, and the object's absolute velocity and compass heading.
      |
      | For more information, please click Help.
      settings: DeleteFcn=PreScanBlockDeleteFcn;
      mask Help: eval('openHelp(462)')
      mask Display:
      | port_label('output',1,'x [m]')
      | port_label('output',2,'y [m]')
      | port_label('output',3,'z [m]','texmode','on')
      | port_label('output',4,'Rotx [deg]','texmode','on')
      | port_label('output',5,'Roty [deg]','texmode','on')
      | port_label('output',6,'Rotz [deg]','texmode','on')
      | port_label('output',7,'GPS lat [deg]','texmode','on')
      | port_label('output',8,'GPS long [deg]','texmode','on')
      | port_label('output',9,'GPS alt [m]','texmode','on')
      | port_label('output',10,'Velocity [m/s]')
      | port_label('output',11,'Heading [deg]')
      | port_label('output',12,'Yaw rate [deg/s]')
  STATE_Audi_A8_1 : Subsystem  Tag=mux/StatePort  Priority=0  LoadFcn=load PrescanStateActuatorData  mask(PreScan Sink Block: State){x0=76.289146423339844, y0=128.47225952148437, z0=0.55, Roll0=0, Pitch0=0, Yaw0=2.5977442419389263E-11, TimeStep=1/100}
      mask prompts: x0 "Ini x-position VEHICLE wrt GLOBAL axis system [m]"; y0 "Ini y-position VEHICLE wrt GLOBAL axis system [m]"; z0 "Ini z-position VEHICLE wrt GLOBAL axis system [m]"; Roll0 "Ini roll-angle BODY wrt VEHICLE axis system [deg]"; Pitch0 "Ini pitch-angle BODY wrt VEHICLE axis system [deg]"; Yaw0 "Ini yaw-angle VEHICLE wrt GLOBAL axis system [deg]"; TimeStep "Auto-Assigned: Upload Period [s]"
      mask help:
      | The Actor State contains a vector signal of size (9x1), containing the following signals:
      |
      | -  Position                  (x,y,z)                                     [m]
      | -  Velocity                  (vx,vy,vz)                               [m/s]
      | -  Angles                    (Roll, Pitch, Yaw)                   [rad]
      |
      | The Actor state is defined in the global axis system.
      | The state is superponed on the Initial position defined in the GUI.
      |
      | For more information, please click Help.
      settings: DeleteFcn=PreScanBlockDeleteFcn;
      mask Help: eval('openHelp(222)')
      mask Display: image(imread('State.png'))
  Scope : Scope
  Selector : Selector  InputPortWidth=5
  State2PathFollowerCnv : Subsystem  Tag=State2PFConnection/cnv
  TIS_2_StandardCoh_Demux : Subsystem  Tag=demux/TIS/StandardCoh  TreatAsAtomicUnit=on  mask(PreScan Demux Block: TIS){MAXMESSAGES=1}
      mask prompts: MAXMESSAGES "Number of Objects"
      mask Help: eval('openHelp(449)')
      mask Display:
      | port_label('input',1,'TIS')
      | port_label('output',1,'Beam ID [-]')
      | port_label('output',2,'Range [m]')
      | port_label('output',3,'DopplerVelocity [m/s]')
      | port_label('output',4,'{\theta} [deg]','texmode','on')
      | port_label('output',5,'{\phi} [deg]','texmode','on')
      | port_label('output',6,'Target ID [-]','texmode','on')
      | port_label('output',7,'TIS Data','texmode','on')
  Terminator_{1..19,21,23} (21 alike) : Terminator
  To Workspace : ToWorkspace  VariableName=Audi_V2V_Data_Recieved  SaveFormat=Timeseries  SampleTime=-1
  Trajectories : Subsystem  Tag=Trajectories  mask(PreScan Source Block: Trajectories){}
      mask help:
      | The Trajectory block contains the trajectories defined in the PreScan Experiment Editor. The output of the trajectory block is the (vehicle) State.
      |
      | For more information, please click Help.
      settings: DeleteFcn=PreScanBlockDeleteFcn;
      mask Help: eval('openHelp(312)')
      mask Display: image(imread('Trajectory.png'));
  Transport Delay{,1..3} (4 alike) : TransportDelay  DelayTime=0.25
  V2X_244_Generic_Expander : Subsystem  LoadFcn=addpath .\V2XPlugin; V2Xbusses;
  V2X_244_Generic_Filter : Subsystem
      mask Display: disp('[1]');
  V2X_Tx244_Generic : Subsystem
  V2X_Tx244_Generic_Enable : Constant  OutDataTypeStr=Inherit: Inherit via back propagation
  pos : Constant  Tag=pos  Value=[76.289146423339844 128.47225952148437 2.5977442419389263E-11]
  STATE_Audi_A8_1_bus : Outport  Tag=outport/StatePort  OutDataTypeStr=Bus: PRESCAN_STATEACTUATORDATA  PortDimensions=1  SampleTime=1/100
  V2X_Tx244_Generic_Transmitter : Outport  Tag=outport/plugin/sfun_V2X_Generic_Transmitter  Port=2
  wires:
  PathFollower_1/2(throttle [%]) -> PPS Model/7(throttle)
  PathFollower_1/3(brake pressure [bar]) -> PPS Model/6(brake dem)
  PPS Model/1(Throttle [%]) -> Dynamics_Simple/2(Throttle)
  PPS Model/2(BrakePres [bar]) -> Dynamics_Simple/3(Brake)
  PPS Model/5(TTC) -> Scope/1
  Dynamics_Simple/3(Perf_Params) -> Bus Selector1/1
  Bus Selector1/1 -> PPS Model/10(RPM)  "<NEngine_[rpm]>"
  Selector/1 -> PPS Model/11(CD)
  [cd] -> Selector/1
  Constant/1 -> PPS Model/8(ind flag)
  MATLAB Function2/3(pedPhi) -> Terminator_21/1
  PPS Model/4(Ped detection flag) -> Terminator_19/1
  SELF_Demux/10(velocity [m/s]) -> [audiVelocity]
  SELF_Demux/1(x [m]) -> [audiX]
  SELF_Demux/2(y [m]) -> [audiY]
  SELF_Demux/6(rotz [deg]) -> [audiRotAngle]
  SELF_Demux/12(yaw rate [deg/s]) -> PPS Model/2(EGO_yaw_rate_[deg/s])
  [audiVelocity] -> PPS Model/1(EGO_velocity [m/s])
  [audiX] -> MATLAB Function2/1(carX)
  [audiY] -> MATLAB Function2/2(carY)
  Constant1/1 -> MATLAB Function2/3(carZ)
  [audiRotAngle] -> MATLAB Function2/4(carRotZ)
  V2X_244_Generic_Filter/1(Filter_Out) -> To Workspace/1, Bus Selector/1
  [audiX] -> MATLAB Function1/1(carX)
  [audiY] -> MATLAB Function1/2(carY)
  Constant2/1 -> MATLAB Function1/3(carZ)
  [audiRotAngle] -> MATLAB Function1/4(carAngle)
  [audiVelocity] -> MATLAB Function1/5(carVelocity)
  Constant3/1 -> MATLAB Function1/12(sensorX)
  Constant4/1 -> MATLAB Function1/13(sensorY)
  Constant5/1 -> MATLAB Function1/14(sensorZ)
  Constant6/1 -> MATLAB Function1/11(dTranslationZ)
  Constant7/1 -> MATLAB Function1/8(pedZ)
  Constant8/1 -> MATLAB Function2/8(sensorCorrX)
  Constant9/1 -> MATLAB Function2/9(sensorCorrY)
  Constant10/1 -> MATLAB Function2/10(sensorCorrZ)
  Constant11/1 -> MATLAB Function2/7(pedZ)
  SELF_Demux/3(z [m]) -> Terminator_23/1
  [pedX] -> MATLAB Function2/5(pedX)
  [pedY] -> MATLAB Function2/6(pedY)
  [pedX] -> MATLAB Function1/6(pedX)
  [pedY] -> MATLAB Function1/7(pedY)
  [pedDTX] -> MATLAB Function1/9(dTranslationX)
  [pedDTY] -> MATLAB Function1/10(dTranslationY)
  Ground_16/1 -> PathFollower_1/2(ActorOffset_Left(+) / Right(-) [m])
  MATLAB Function/1(pedR_Array) -> PPS Model/3(TIS_range [m])
  MATLAB Function/3(dVel_Array) -> PPS Model/4(TIS_rangedot [m/s])
  MATLAB Function/2(pedTheta_Array) -> PPS Model/5(TIS_theta [deg])
  STATE_Audi_A8_1/1(StateBus) -> STATE_Audi_A8_1_bus/1, [State]
  SELF_Audi_A8_1/1 -> SELF_Demux/1(SELF)
  CameraSensor_1/1 -> CameraSensor_1_MM_Demux/1(In1)
  CameraSensor_1_MM_Demux/1(I) -> CameraSensor_1_MM_Display/1
  TIS_2/1 -> TIS_2_StandardCoh_Demux/1(TIS)
  pos/1 -> PathFollower_1/1(TrajOffset_x,y,Y [m,m,deg])
  InitialVelocity/1 -> PathFollower_1/4(Initial Velocity [m/s])
  DesiredVelocity/1 -> PathFollower_1/5(Desired Velocity [m/s])
  [State] -> State2PathFollowerCnv/1(State BUS)
  State2PathFollowerCnv/2(velocity [m/s]) -> PathFollower_1/6(velocity [m/s])
  State2PathFollowerCnv/3(position x,y,Y [m,m,deg]) -> PathFollower_1/3(position x,y,Y [m,m,deg])
  PathFollower_1/1(delta_steerwheel [deg]) -> Dynamics_Simple/1(DeltaSteer_[deg])
  PathFollower_1/4(v0 [m/s]) -> Dynamics_Simple/4(Initial_Vx_[ms-1])
  PathFollower_1/5(Auto_GearShift) -> Dynamics_Simple/6(Auto_GearShift)
  Dynamics_Simple/1(State) -> STATE_Audi_A8_1/1(State)
  V2X_Tx244_Generic_Enable/1 -> V2X_Tx244_Generic/1(Enabled)
  V2X_Tx244_Generic/1(PRESCAN_V2X_USER_GENERIC_MESSAGE) -> V2X_244_Generic_Expander/1(In)
  V2X_244_Generic_Expander/1(Out) -> V2X_Tx244_Generic_Transmitter/1
  V2X_Rx244_Generic_Receiver/1 -> V2X_244_Generic_Filter/1(Filter_In)
  Ground_1/1 -> Dynamics_Simple/5(AutoManual_OnOff)
  Ground_2/1 -> Dynamics_Simple/7(Manual_GearShift)
  Dynamics_Simple/2(Vx [m s-1]) -> Terminator_1/1
  Ground_3/1 -> PPS Model/9(img)
  PathFollower_1/6(Actor/Traj_distance [m]) -> Terminator_2/1
  PathFollower_1/7(Actor/Traj_angle [deg]) -> Terminator_3/1
  SELF_Demux/4(rotx [deg]) -> Terminator_4/1
  SELF_Demux/5(roty [deg]) -> Terminator_5/1
  SELF_Demux/7(GPS lat [deg]) -> Terminator_6/1
  SELF_Demux/8(GPS long [deg]) -> Terminator_7/1
  SELF_Demux/9(GPS alt [m]) -> Terminator_8/1
  SELF_Demux/11(heading [deg]) -> Terminator_9/1
  State2PathFollowerCnv/1(Yaw rate [deg/s]) -> Terminator_10/1
  TIS_2_StandardCoh_Demux/1(Out1) -> Terminator_11/1
  TIS_2_StandardCoh_Demux/2(Out2) -> Terminator_12/1
  TIS_2_StandardCoh_Demux/3(Out3) -> Terminator_13/1
  TIS_2_StandardCoh_Demux/4(Out4) -> Terminator_14/1
  TIS_2_StandardCoh_Demux/5(Out5) -> Terminator_15/1
  TIS_2_StandardCoh_Demux/6(Out7) -> Terminator_16/1
  TIS_2_StandardCoh_Demux/7(Out6) -> Terminator_17/1
  Trajectories/1(State) -> Terminator_18/1
  Ground_4/1 -> V2X_Tx244_Generic/2(DATA.messageID)
  Ground_5/1 -> V2X_Tx244_Generic/3(DATA.senderID)
  Ground_6/1 -> V2X_Tx244_Generic/4(DATA.signal_1)
  Ground_7/1 -> V2X_Tx244_Generic/5(DATA.signal_2)
  Ground_8/1 -> V2X_Tx244_Generic/6(DATA.signal_3)
  Ground_9/1 -> V2X_Tx244_Generic/7(DATA.signal_4)
  Ground_10/1 -> V2X_Tx244_Generic/8(DATA.signal_5)
  Ground_11/1 -> V2X_Tx244_Generic/9(DATA.signal_6)
  Ground_12/1 -> V2X_Tx244_Generic/10(DATA.signal_7)
  Ground_13/1 -> V2X_Tx244_Generic/11(DATA.signal_8)
  Ground_14/1 -> V2X_Tx244_Generic/12(DATA.signal_9)
  Ground_15/1 -> V2X_Tx244_Generic/13(DATA.signal_10)
  MATLAB Function2/1(pedR) -> MATLAB Function/1(pedR)
  MATLAB Function2/2(pedTheta) -> MATLAB Function/2(pedTheta)
  MATLAB Function1/1(dopplerVelocity) -> MATLAB Function/3(dVel)
  Transport Delay/1 -> [pedX]
  Transport Delay1/1 -> [pedY]
  Transport Delay2/1 -> [pedDTX]
  Transport Delay3/1 -> [pedDTY]
  Bus Selector/1 -> Transport Delay/1  "<signal_1>"
  Bus Selector/2 -> Transport Delay1/1  "<signal_2>"
  Bus Selector/3 -> Transport Delay2/1  "<signal_3>"
  Bus Selector/4 -> Transport Delay3/1  "<signal_4>"
